simulink model "Project_Vehicle_Model_Round_Two"  (R2021b)
settings: Solver=VariableStepAuto  StartTime=0  StopTime=1923  MaxStep=0.01  RelTol=1e-3
values from neighbouring files (symbols this model uses):
  A_CS = 12    [Project_Round_Two.m]
  battery_cell_p = 6    [QSS_simulation.m]
  battery_cell_s = cell_nbr(i_k)    [QSS_simulation.m]
  battery_file_name = 'init_Kokam_BT'    [QSS_simulation.m]
  battery_init_soc = soc_final    (= 0.9)    [QSS_simulation.m]
  C_D = 0.36    [Project_Round_Two.m]
  F_RR = round(f_RR * mass_total * g * cos(beta))    [Project_Round_Two.m]
  F_slope = round(mass_total * g * sin(beta))    [Project_Round_Two.m]
  gear_ratio = 5    [Project_Round_Two.m]
  mass_total = round(mass_veh + mass_payload +               mass_batt + mass_motor)    [Project_Round_Two.m]
  P_aux = 10    [Project_Round_Two.m]
  RHO = 1.17    [Project_Round_Two.m]
  speed_m_s = speed_km_h .* (5/18)    [Project_Round_Two.m]
  trans_eff = 0.9    [Project_Round_Two.m]
  tyre_dyn_r = tyre_dyn_d/2    (= 0.34325)    [Project_Round_Two.m]
undefined symbols (not defined in the file or in its folder): cap_BT, DiscIntNeverNeededParam, eta_EM_map, rchg_map_BT, rdis_map_BT, soc_map_BT, T_EM_max, voc_map_BT, w_EM_row, w_EM_upper
libraries: slpidlib x1
settings Model: Creator=tammik2  LastModifiedBy=User
settings SolverCC: ZeroCrossAlgorithm=Adaptive  AlgebraicLoopSolver=TrustRegion
settings DataIOCC: ReturnWorkspaceOutputs=off
settings DebuggingCC: IgnoredZcDiagnostic=none  SFMachineParentedDataDiag=warning  ArithmeticOperatorsInVariantConditions=warning
settings SFSimCC: SimUseLocalCustomCode=off  CustomCodeUndefinedFunction=UseInterfaceOnly
settings RTWCC: RTWUseLocalCustomCode=off
settings CodeAppCC: StateflowObjectComments=on

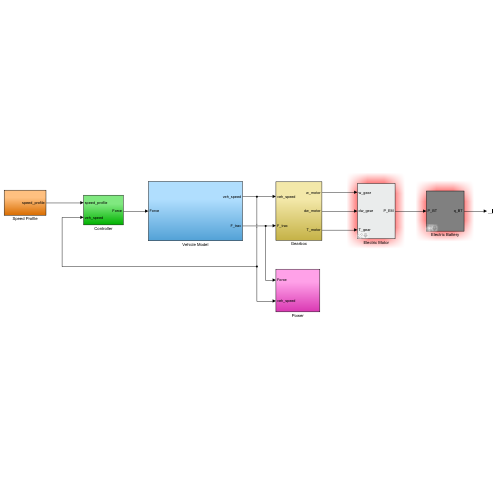
[thumbnail: Simulink's stored preview of the top-level diagram]
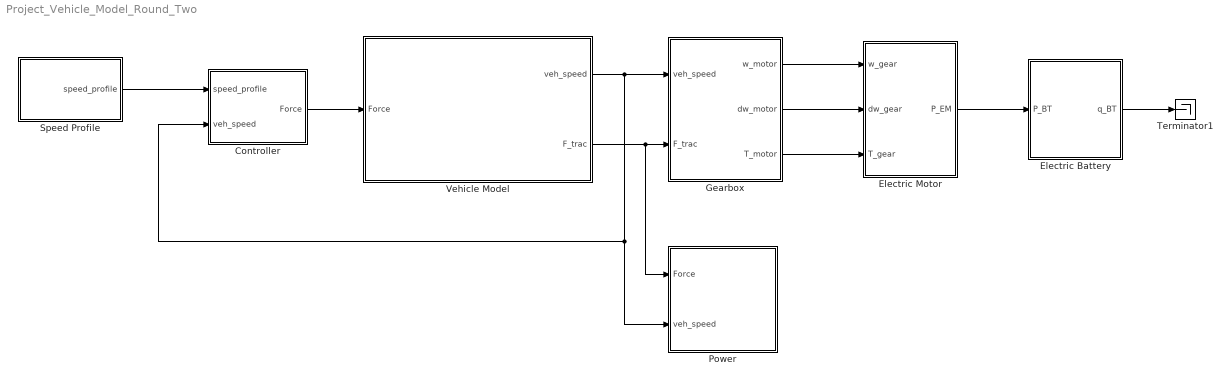
== system Project_Vehicle_Model_Round_Two ==
  Controller : Subsystem
  Electric Battery : Subsystem  Tag=battery  AncestorBlock=qss_tb_library_aalto/Energy Buffer/Battery v3  mask(Battery){init_soc_BT=battery_init_soc, cell_series_BT=battery_cell_s, cell_parallel_BT=battery_cell_p, init_file_BT=battery_file_name}
      mask prompts: init_soc_BT "Initial charge of battery"; cell_series_BT "Cells in series"; cell_parallel_BT "Cells in parallel"; init_file_BT "Battery initialization file"
      mask init:
      | eval(init_file_BT)
  Electric Motor : Subsystem  AncestorBlock=qss_tb_library_aalto/Energy Converter/Electric Motor v2  mask(Electric Motor){scale_EM=3.5, theta_EM=0.5, P_aux=P_aux*1000, over_factor=1.25}
      mask prompts: scale_EM "Motor scaling factor [-]"; theta_EM "Motor inertia [kg*m2]"; P_aux "Power required by auxiliaries [W]"; over_factor "Overtorque factor"
      mask help:
      | This block simulates the behaviour of an electric motor. The block is based on an efficiency map.
      |
      | Input:
      | =====
      | 	w_gear		Speed of the fly wheel [rad/s]
      | 	dw_gear	Acceleration of the fly wheel [rad/s^2]
      | 	T_gear		Torque on the fly wheel [Nm]
      |
      | Output:
      | ======
      | 	P_EM		Power produced by the electric motor [W]
      mask init:
      | init_EM;
  Gearbox : Subsystem
  Power : Subsystem
  Speed Profile : Subsystem
  Terminator1 : Terminator
  Vehicle Model : Subsystem
  wires:
  Controller/1(Force) -> Vehicle Model/1(Force)
  Speed Profile/1(speed_profile) -> Controller/1(speed_profile)
  Electric Battery/1(q_BT) -> Terminator1/1
  Vehicle Model/2(F_trac) -> Power/1(Force), Gearbox/2(F_trac)
  Vehicle Model/1(veh_speed) -> Controller/2(veh_speed), Power/2(veh_speed), Gearbox/1(veh_speed)
  Gearbox/1(w_motor) -> Electric Motor/1(w_gear)
  Gearbox/2(dw_motor) -> Electric Motor/2(dw_gear)
  Gearbox/3(T_motor) -> Electric Motor/3(T_gear)
  Electric Motor/1(P_EM) -> Electric Battery/1(P_BT)

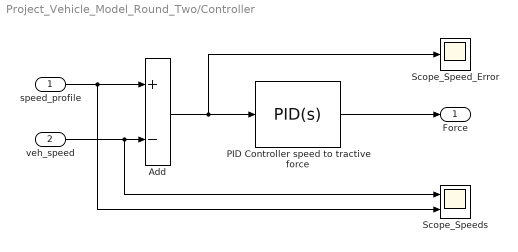
== system Project_Vehicle_Model_Round_Two/Controller ==
  speed_profile : Inport
  veh_speed : Inport  Port=2
  Add : Sum  Inputs=+-
  PID Controller speed to tractive force : slpidlib/PID Controller  Controller=PID  Form=Parallel  TimeDomain=Continuous-time  UseExternalTs=off  SampleTime=-1  IntegratorMethod=Forward Euler  FilterMethod=Forward Euler  ControllerParametersSource=internal  P=21430.8579873667  I=4099.34459462088  D=-4516.26276730351  UseFilter=on  N=1.72044274974478  TunerSelectOption=Transfer Function Based (PID Tuner App)  InitialConditionSource=internal  InitialConditionForIntegrator=0  InitialConditionForFilter=0  DifferentiatorICPrevScaledInput=0  ExternalReset=none  TrackingMode=off  Kt=1  LimitOutput=off  SatLimitsSource=internal  UpperSaturationLimit=inf  LowerSaturationLimit=-inf  LinearizeAsGain=on  AntiWindupMode=none  Kb=1  POutMin=[]  POutMax=[]  IOutMin=[]  IOutMax=[]  DOutMin=[]  DOutMax=[]  NOutMin=[]  NOutMax=[]  SumOutMin=[]  SumOutMax=[]  SaturationOutMin=[]  SaturationOutMax=[]  PParamMin=[]  PParamMax=[]  IParamMin=[]  IParamMax=[]  DParamMin=[]  DParamMax=[]  NParamMin=[]  NParamMax=[]  KbParamMin=[]  KbParamMax=[]  KtParamMin=[]  KtParamMax=[]  KbOutMin=[]  KbOutMax=[]  KtOutMin=[]  KtOutMax=[]  IntegratorOutMin=[]  IntegratorOutMax=[]  FilterOutMin=[]  FilterOutMax=[]  SumI1OutMin=[]  SumI1OutMax=[]  SumI2OutMin=[]  SumI2OutMax=[]  SumI3OutMin=[]  SumI3OutMax=[]  SumI4OutMin=[]  SumI4OutMax=[]  SumDOutMin=[]  SumDOutMax=[]  DifferentiatorOutMin=[]  DifferentiatorOutMax=[]  FilterDiffOutCoefMin=[]  FilterDiffOutCoefMax=[]  ReciprocalOutMin=[]  ReciprocalOutMax=[]  SumDenOutMin=[]  SumDenOutMax=[]  SumNumOutMin=[]  SumNumOutMax=[]  DivideOutMin=[]  DivideOutMax=[]  UdiffTsProdOutMin=[]  UdiffTsProdOutMax=[]  NTsProdOutMin=[]  NTsProdOutMax=[]  UintegralTsProdOutMin=[]  UintegralTsProdOutMax=[]  UngainTsProdOutMin=[]  UngainTsProdOutMax=[]  IntegratorContinuousStateAttributes=''  IntegratorStateMustResolveToSignalObject=off  IntegratorRTWStateStorageClass=Auto  FilterContinuousStateAttributes=''  FilterStateMustResolveToSignalObject=off  FilterRTWStateStorageClass=Auto  ParallelPVariant=InternalParameters  IdealPVariant=Disabled  IVariant=InternalParameters  DVariant=InternalParameters  IntegratorVariant=Continuous  SatVariant=Disabled  AWVariant=Passthrough  PCopyVariant=Disabled  TRVariant=Disabled  FdbkBlocksVariant=Forward  IdealPFdbkVariant=Disabled  SatFdbkVariant=Disabled  DerivativeFilterVariant=ContFilter  NVariant=InternalParameters  NCopyVariant=Disabled  FilterICVariant=InternalICsFilter  IntegratorICVariant=InternalICs  ExternalResetVariant=Disabled  TRSumVariant=Passthrough  SumFdbkVariant=Disabled  SumVariant=Sum_PID  TsampFilterVariant=InternalTs  TsampNgainVariant=Passthrough  TsampIntegralVariant=Passthrough  ExternalSaturationOutDataTypeStr=Inherit: Same as second input
  "Scope_Speed_Error " : Scope
  Scope_Speeds : Scope  NumInputPorts=2
  Force : Outport  VectorParamsAs1DForOutWhenUnconnected=off
  wires:
  veh_speed/1 -> Scope_Speeds/1, Add/2
  speed_profile/1 -> Scope_Speeds/2, Add/1
  Add/1 -> "Scope_Speed_Error "/1, PID Controller speed to tractive force/1
  PID Controller speed to tractive force/1 -> Force/1

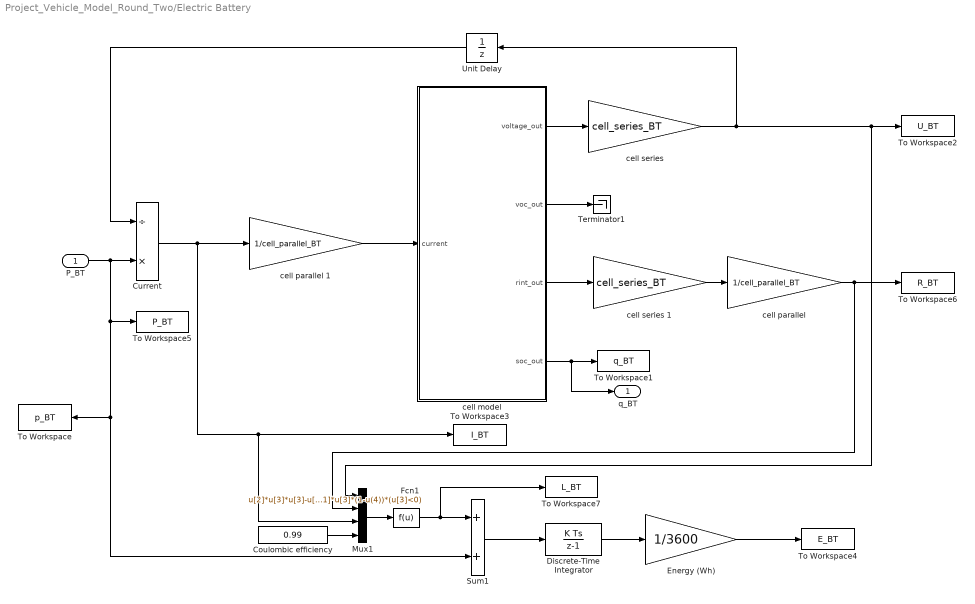
== system Project_Vehicle_Model_Round_Two/Electric Battery ==
  P_BT : Inport
  Coulombic efficiency : Constant  Value=0.99
  Current : Product  Inputs=/*  RndMeth=Zero
  Discrete-Time Integrator : DiscreteIntegrator  ICPrevOutput=DiscIntNeverNeededParam  ICPrevScaledInput=DiscIntNeverNeededParam
  Energy (Wh) : Gain  Gain=1/3600
  Fcn1 : Fcn  Expr=u[2]*u[3]*u[3]-u[1]*u[3]*(1-u(4))*(u[3]<0)
  Mux1 : Mux
  Sum1 : Sum  InputSameDT=on  SaturateOnIntegerOverflow=on  OutDataTypeStr=Inherit: Same as first input
  Terminator1 : Terminator
  To Workspace : ToWorkspace  VariableName=p_BT  SaveFormat=Timeseries  SampleTime=-1
  To Workspace1 : ToWorkspace  VariableName=q_BT  SampleTime=-1
  To Workspace2 : ToWorkspace  VariableName=U_BT  SampleTime=-1
  To Workspace3 : ToWorkspace  VariableName=I_BT  SampleTime=-1
  To Workspace4 : ToWorkspace  VariableName=E_BT  SampleTime=-1
  To Workspace5 : ToWorkspace  VariableName=P_BT  SampleTime=-1
  To Workspace6 : ToWorkspace  VariableName=R_BT  SampleTime=-1
  To Workspace7 : ToWorkspace  VariableName=L_BT  SampleTime=-1
  Unit Delay : UnitDelay  InitialCondition=cell_series_BT*max(voc_map_BT)  SampleTime=-1  HasFrameUpgradeWarning=on
  cell model : Subsystem
  cell parallel : Gain  Gain=1/cell_parallel_BT
  cell parallel 1 : Gain  Gain=1/cell_parallel_BT
  "cell series " : Gain  Gain=cell_series_BT
  cell series 1 : Gain  Gain=cell_series_BT
  q_BT : Outport  InitialOutput=0  VectorParamsAs1DForOutWhenUnconnected=off
  wires:
  cell model/1(voltage_out) -> "cell series "/1
  "cell series "/1 -> Unit Delay/1, To Workspace2/1, Mux1/1
  cell model/3(rint_out) -> cell series 1/1
  cell series 1/1 -> cell parallel/1
  P_BT/1 -> Current/2, To Workspace5/1, To Workspace/1, Sum1/2
  cell model/2(voc_out) -> Terminator1/1
  Unit Delay/1 -> Current/1
  Current/1 -> cell parallel 1/1, To Workspace3/1, Mux1/3
  cell model/4(soc_out) -> To Workspace1/1, q_BT/1
  cell parallel/1 -> To Workspace6/1, Mux1/2
  cell parallel 1/1 -> cell model/1(current)
  Discrete-Time Integrator/1 -> Energy (Wh)/1
  Fcn1/1 -> Sum1/1, To Workspace7/1
  Sum1/1 -> Discrete-Time Integrator/1
  Energy (Wh)/1 -> To Workspace4/1
  Mux1/1 -> Fcn1/1
  Coulombic efficiency/1 -> Mux1/4

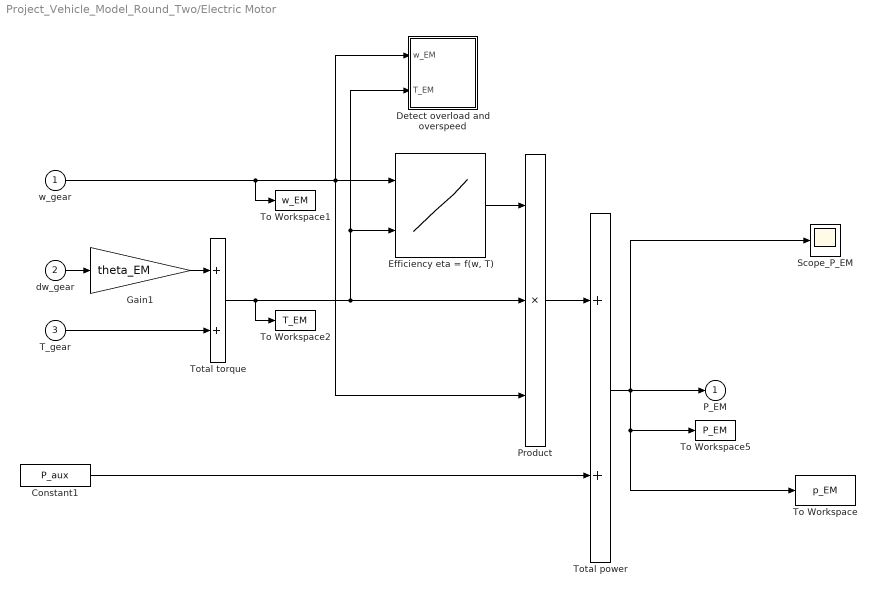
== system Project_Vehicle_Model_Round_Two/Electric Motor ==
  w_gear : Inport
  dw_gear : Inport  Port=2
  T_gear : Inport  Port=3
  Constant1 : Constant  Value=P_aux
  Detect overload and overspeed : Subsystem
  "Efficiency eta = f(w, T)" : Lookup2D  RowIndex=w_EM_row  ColumnIndex=T_EM_col  Table=eta_EM_map
  Gain1 : Gain  Gain=theta_EM  SaturateOnIntegerOverflow=on  OutDataTypeStr=Inherit: Same as input  ParamDataTypeStr=Inherit: Same as input
  Product : Product  Inputs=3  InputSameDT=on  RndMeth=Zero  SaturateOnIntegerOverflow=on  OutDataTypeStr=Inherit: Same as first input
  Scope_P_EM : Scope
  To Workspace : ToWorkspace  VariableName=p_EM  SaveFormat=Timeseries  SampleTime=-1
  To Workspace1 : ToWorkspace  VariableName=w_EM  SampleTime=-1
  To Workspace2 : ToWorkspace  VariableName=T_EM  SampleTime=-1
  To Workspace5 : ToWorkspace  VariableName=P_EM  SampleTime=-1
  Total power : Sum  InputSameDT=on  SaturateOnIntegerOverflow=on  OutDataTypeStr=Inherit: Same as first input
  Total torque : Sum  InputSameDT=on  SaturateOnIntegerOverflow=on  OutDataTypeStr=Inherit: Same as first input
  P_EM : Outport  InitialOutput=0  VectorParamsAs1DForOutWhenUnconnected=off
  wires:
  w_gear/1 -> Detect overload and overspeed/1(w_EM), "Efficiency eta = f(w, T)"/1, Product/3, To Workspace1/1
  "Efficiency eta = f(w, T)"/1 -> Product/1
  dw_gear/1 -> Gain1/1
  T_gear/1 -> Total torque/2
  Gain1/1 -> Total torque/1
  Total torque/1 -> Detect overload and overspeed/2(T_EM), "Efficiency eta = f(w, T)"/2, Product/2, To Workspace2/1
  Constant1/1 -> Total power/2
  Product/1 -> Total power/1
  Total power/1 -> Scope_P_EM/1, P_EM/1, To Workspace5/1, To Workspace/1

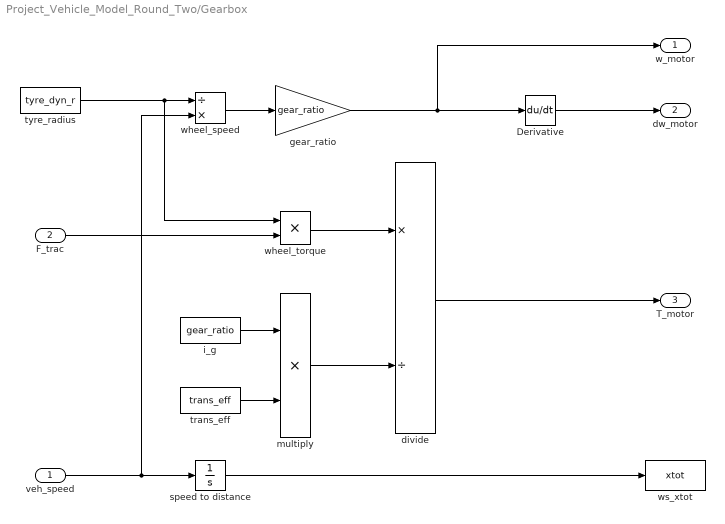
== system Project_Vehicle_Model_Round_Two/Gearbox ==
  veh_speed : Inport
  F_trac : Inport  Port=2
  Derivative : Derivative
  divide : Product  Inputs=*/
  gear_ratio : Gain  Gain=gear_ratio
  i_g : Constant  Value=gear_ratio
  multiply : Product  Inputs=**
  speed to distance : Integrator
  trans_eff : Constant  Value=trans_eff
  tyre_radius : Constant  Value=tyre_dyn_r
  wheel_speed : Product  Inputs=/*
  wheel_torque : Product  Inputs=**
  ws_xtot : ToWorkspace  VariableName=xtot  SaveFormat=Timeseries  SampleTime=-1
  w_motor : Outport  VectorParamsAs1DForOutWhenUnconnected=off
  dw_motor : Outport  Port=2  VectorParamsAs1DForOutWhenUnconnected=off
  T_motor : Outport  Port=3  VectorParamsAs1DForOutWhenUnconnected=off
  wires:
  tyre_radius/1 -> wheel_torque/1, wheel_speed/1
  wheel_speed/1 -> gear_ratio/1
  gear_ratio/1 -> Derivative/1, w_motor/1
  wheel_torque/1 -> divide/1
  multiply/1 -> divide/2
  i_g/1 -> multiply/1
  trans_eff/1 -> multiply/2
  divide/1 -> T_motor/1
  Derivative/1 -> dw_motor/1
  veh_speed/1 -> wheel_speed/2, speed to distance/1
  F_trac/1 -> wheel_torque/2
  speed to distance/1 -> ws_xtot/1

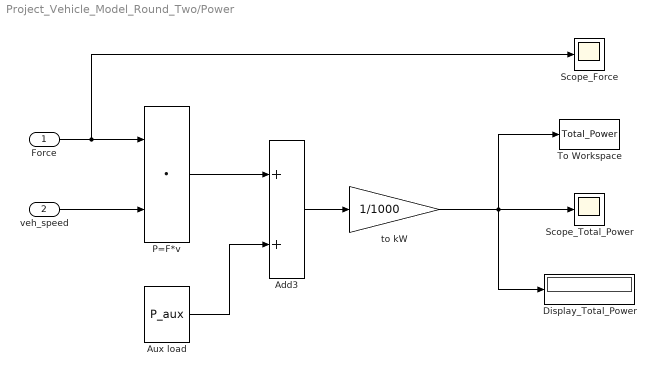
== system Project_Vehicle_Model_Round_Two/Power ==
  Force : Inport
  veh_speed : Inport  Port=2
  Add3 : Sum
  Aux load : Constant  Value=P_aux
  Display_Total_Power : Display
  P=F*v : DotProduct  InputSameDT=on  OutDataTypeStr=Inherit: Inherit via internal rule
  Scope_Force : Scope
  Scope_Total_Power : Scope
  To Workspace : ToWorkspace  VariableName=Total_Power  SaveFormat=Timeseries  SampleTime=-1
  to kW : Gain  Gain=1/1000
  wires:
  veh_speed/1 -> P=F*v/2
  Force/1 -> Scope_Force/1, P=F*v/1
  P=F*v/1 -> Add3/1
  Aux load/1 -> Add3/2
  Add3/1 -> to kW/1
  to kW/1 -> Display_Total_Power/1, To Workspace/1, Scope_Total_Power/1

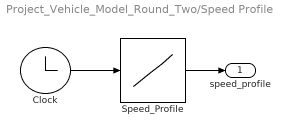
== system Project_Vehicle_Model_Round_Two/Speed Profile ==
  Clock : Clock
  Speed_Profile : Lookup_n-D  NumberOfTableDimensions=1  BreakpointsSpecification=Even spacing  BreakpointsForDimension1=[0:1923]  Table=speed_m_s  InternalRulePriority=Speed  RndMeth=Simplest  InputSameDT=on
  speed_profile : Outport  VectorParamsAs1DForOutWhenUnconnected=off
  wires:
  Clock/1 -> Speed_Profile/1
  Speed_Profile/1 -> speed_profile/1

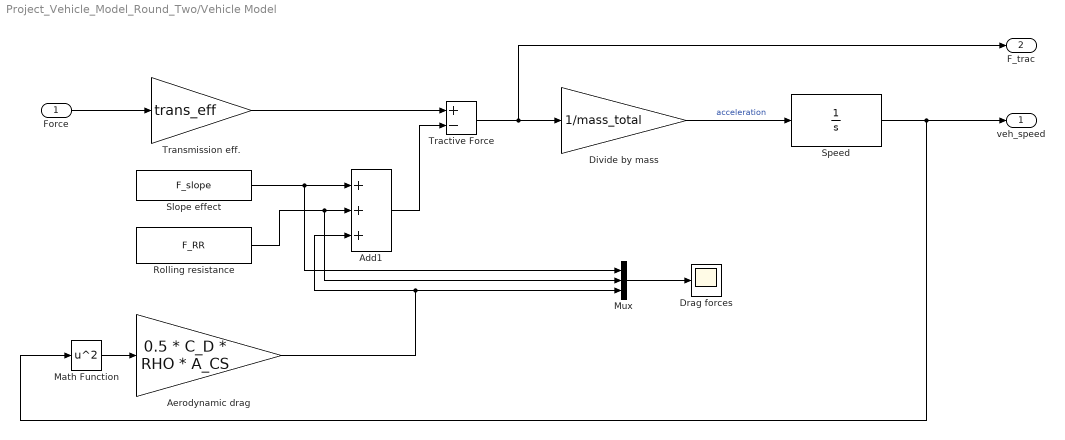
== system Project_Vehicle_Model_Round_Two/Vehicle Model ==
  Force : Inport
  Add1 : Sum  Inputs=+++
  Aerodynamic drag : Gain  Gain=0.5 * C_D * RHO * A_CS
  "Divide by mass " : Gain  Gain=1/mass_total
  Drag forces : Scope
  Math Function : Math  Operator=square  SignedPower=on  SaturateOnIntegerOverflow=on
  Mux : Mux  Inputs=3
  Rolling resistance : Constant  Value=F_RR
  Slope effect : Constant  Value=F_slope
  Speed : TransferFcn  Denominator=[1 0]
  Tractive Force : Sum  Inputs=+-
  Transmission eff. : Gain  Gain=trans_eff
  veh_speed : Outport  VectorParamsAs1DForOutWhenUnconnected=off
  F_trac : Outport  Port=2  VectorParamsAs1DForOutWhenUnconnected=off
  wires:
  Speed/1 -> Math Function/1, veh_speed/1
  Force/1 -> Transmission eff./1
  Rolling resistance/1 -> Mux/2, Add1/2
  "Divide by mass "/1 -> Speed/1  "acceleration"
  Add1/1 -> Tractive Force/2
  Math Function/1 -> Aerodynamic drag/1
  Transmission eff./1 -> Tractive Force/1
  Aerodynamic drag/1 -> Add1/3, Mux/3
  Mux/1 -> Drag forces/1
  Tractive Force/1 -> F_trac/1, "Divide by mass "/1
  Slope effect/1 -> Mux/1, Add1/1

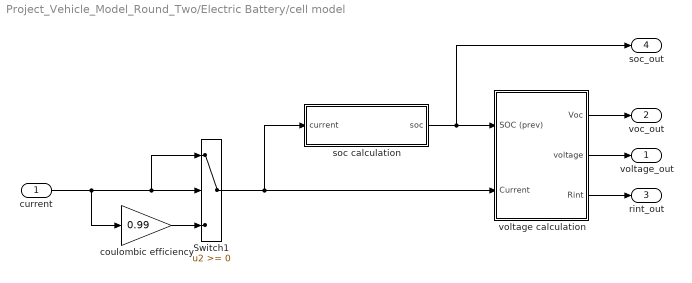
== system Project_Vehicle_Model_Round_Two/Electric Battery/cell model ==
  current : Inport
  Switch1 : Switch  SaturateOnIntegerOverflow=on  InputSameDT=on
  coulombic efficiency : Gain  Gain=0.99
  soc calculation : Subsystem
  voltage calculation : Subsystem
  voltage_out : Outport  VectorParamsAs1DForOutWhenUnconnected=off
  voc_out : Outport  Port=2  VectorParamsAs1DForOutWhenUnconnected=off
  rint_out : Outport  Port=3  VectorParamsAs1DForOutWhenUnconnected=off
  soc_out : Outport  Port=4  VectorParamsAs1DForOutWhenUnconnected=off
  wires:
  Switch1/1 -> soc calculation/1(current), voltage calculation/2(Current)
  current/1 -> Switch1/2, Switch1/1, coulombic efficiency/1
  coulombic efficiency/1 -> Switch1/3
  voltage calculation/3(Rint) -> rint_out/1
  voltage calculation/1(Voc) -> voc_out/1
  voltage calculation/2(voltage) -> voltage_out/1
  soc calculation/1(soc) -> voltage calculation/1(SOC (prev)), soc_out/1

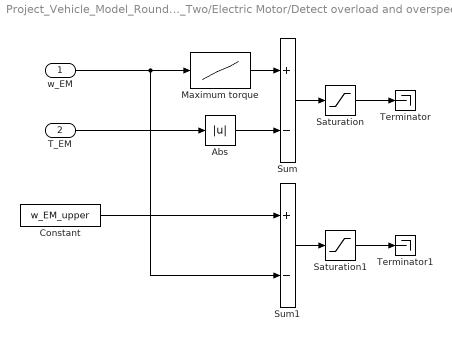
== system Project_Vehicle_Model_Round_Two/Electric Motor/Detect overload and overspeed ==
  w_EM : Inport
  T_EM : Inport  Port=2
  Abs : Abs  SaturateOnIntegerOverflow=on
  Constant : Constant  Value=w_EM_upper
  Maximum torque : Lookup  InputValues=w_EM_row  Table=T_EM_max*over_factor  SaturateOnIntegerOverflow=on
  Saturation : Saturate  UpperLimit=0  LowerLimit=-inf
  Saturation1 : Saturate  UpperLimit=0  LowerLimit=-inf
  Sum : Sum  Inputs=+-  InputSameDT=on  SaturateOnIntegerOverflow=on  OutDataTypeStr=Inherit: Same as first input
  Sum1 : Sum  Inputs=+-  InputSameDT=on  SaturateOnIntegerOverflow=on  OutDataTypeStr=Inherit: Same as first input
  Terminator : Terminator
  Terminator1 : Terminator
  wires:
  Saturation1/1 -> Terminator1/1
  Sum1/1 -> Saturation1/1
  Constant/1 -> Sum1/1
  Saturation/1 -> Terminator/1
  Abs/1 -> Sum/2
  Maximum torque/1 -> Sum/1
  T_EM/1 -> Abs/1
  w_EM/1 -> Sum1/2, Maximum torque/1
  Sum/1 -> Saturation/1

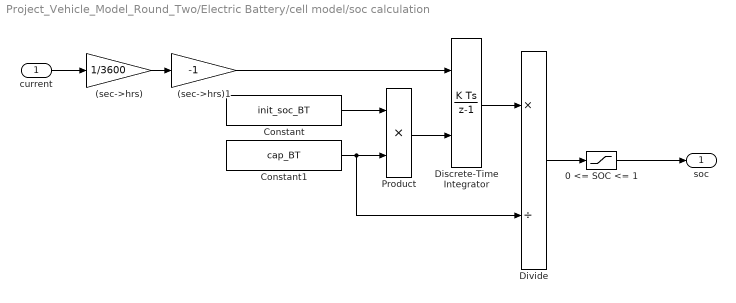
== system Project_Vehicle_Model_Round_Two/Electric Battery/cell model/soc calculation ==
  current : Inport
  (sec->hrs) : Gain  Gain=1/3600  SaturateOnIntegerOverflow=on  OutDataTypeStr=Inherit: Same as input  ParamDataTypeStr=Inherit: Same as input
  (sec->hrs)1 : Gain  Gain=-1  SaturateOnIntegerOverflow=on  OutDataTypeStr=Inherit: Same as input  ParamDataTypeStr=Inherit: Same as input
  0 <= SOC <= 1 : Saturate  UpperLimit=1  LowerLimit=0
  Constant : Constant  Value=init_soc_BT
  Constant1 : Constant  Value=cap_BT
  Discrete-Time Integrator : DiscreteIntegrator  InitialConditionSource=external  ICPrevOutput=DiscIntNeverNeededParam  ICPrevScaledInput=DiscIntNeverNeededParam
  Divide : Product  Inputs=*/  RndMeth=Zero
  Product : Product  RndMeth=Zero
  soc : Outport  VectorParamsAs1DForOutWhenUnconnected=off
  wires:
  current/1 -> (sec->hrs)/1
  0 <= SOC <= 1/1 -> soc/1
  (sec->hrs)/1 -> (sec->hrs)1/1
  Discrete-Time Integrator/1 -> Divide/1
  Divide/1 -> 0 <= SOC <= 1/1
  Constant/1 -> Product/1
  Product/1 -> Discrete-Time Integrator/2
  (sec->hrs)1/1 -> Discrete-Time Integrator/1
  Constant1/1 -> Product/2, Divide/2

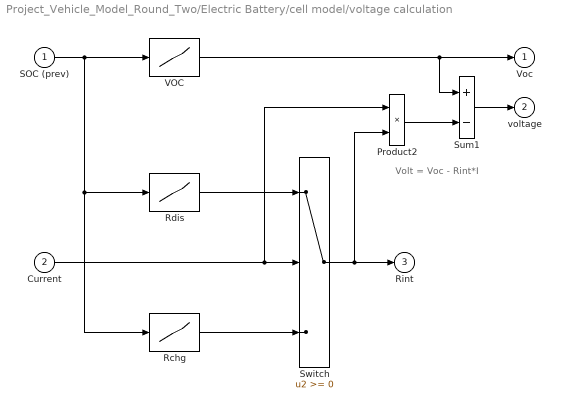
== system Project_Vehicle_Model_Round_Two/Electric Battery/cell model/voltage calculation ==
  note: Volt = Voc - Rint*I
  SOC (prev) : Inport
  Current : Inport  Port=2
  Product2 : Product  InputSameDT=on  SaturateOnIntegerOverflow=on  OutDataTypeStr=Inherit: Same as first input
  Rchg : Lookup  InputValues=soc_map_BT  Table=rchg_map_BT  SaturateOnIntegerOverflow=on
  Rdis : Lookup  InputValues=soc_map_BT  Table=rdis_map_BT  SaturateOnIntegerOverflow=on
  Sum1 : Sum  Inputs=+-  InputSameDT=on  SaturateOnIntegerOverflow=on  OutDataTypeStr=Inherit: Same as first input
  Switch : Switch  SaturateOnIntegerOverflow=on  InputSameDT=on
  VOC : Lookup  InputValues=soc_map_BT  Table=voc_map_BT  SaturateOnIntegerOverflow=on
  Voc : Outport  InitialOutput=0  VectorParamsAs1DForOutWhenUnconnected=off
  voltage : Outport  Port=2  InitialOutput=0  VectorParamsAs1DForOutWhenUnconnected=off
  Rint : Outport  Port=3  InitialOutput=0  VectorParamsAs1DForOutWhenUnconnected=off
  wires:
  Switch/1 -> Rint/1, Product2/2
  Rdis/1 -> Switch/1
  Rchg/1 -> Switch/3
  VOC/1 -> Voc/1, Sum1/1
  SOC (prev)/1 -> VOC/1, Rdis/1, Rchg/1
  Product2/1 -> Sum1/2
  Sum1/1 -> voltage/1
  Current/1 -> Switch/2, Product2/1
